simulink model "USART_1_Receive_Send"  (R2018b)
settings: Solver=FixedStepDiscrete  StartTime=0.0  StopTime=10  FixedStep=0.5  RelTol=1e-3  EnableMultiTasking=on
libraries: USART_Lib x6, STM32_Config_Lib x1
settings Model: Creator=reynaudp  LastModifiedBy=bannou
settings DataIOCC: LimitDataPoints=on  SaveFormat=Array  SignalLoggingSaveFormat=ModelDataLogs
settings OptimizationCC: DefaultParameterBehavior=Inlined  DefaultUnderspecifiedDataType=single  LifeSpan=1
settings DebuggingCC: UnderspecifiedInitializationDetection=Classic  MergeDetectMultiDrivingBlocksExec=none  SolverPrmCheckMsg=warning  MultiTaskDSMMsg=warning  MultiTaskCondExecSysMsg=none  AllowSymbolicDim=off  SFUnexpectedBacktrackingDiag=warning  SFNoUnconditionalDefaultTransitionDiag=warning  SFExecutionAtInitializationDiag=none
settings HardwareCC: ProdBitPerPointer=32  ProdBitPerSizeT=32  ProdBitPerPtrDiffT=32  ProdLargestAtomicInteger=Integer  ProdWordSize=32  ProdHWDeviceType=STMicroelectronics->STM32 32-bit Cortex-M
settings ModelReferenceCC: PropagateSignalLabelsOutOfModel=off
settings SFSimCC: SimUseLocalCustomCode=off  CompileTimeRecursionLimit=0  MATLABDynamicMemAlloc=off
settings RTWCC: SystemTargetFile=stm32.tlc  TemplateMakefile=stm32.tmf  Description=stm32 (Embedded Target)  RTWUseLocalCustomCode=off
settings CodeAppCC: IgnoreCustomStorageClasses=off  SimulinkDataObjDesc=on  CustomSymbolStrType=$N$R$M  InsertBlockDesc=on
settings STFCustomTargetCC: CodeReplacementLibrary=ARM CMSIS SIN COS  ParMdlRefBuildCompliant=on  IncludeMdlTerminateFcn=off  CombineOutputUpdateFcns=on  ERTCustomFileBanners=on  SupportNonFinite=off  SupportComplex=off  SupportContinuousTime=off  SupportNonInlinedSFcns=off  RemoveResetFunc=on  SupportVariableSizeSignals=on  MATLABClassNameForMDSCustomization=Simulink.SoftwareTarget.ERTCustomization  SystemTargetFile=stm32.tlc
settings ERTTargetCC: CodeReplacementLibrary=ARM CMSIS SIN COS  MultiwordLength=2048  CompOptLevelCompliant=off  ConcurrentExecutionCompliant=off  IncludeMdlTerminateFcn=off  SupportNonFinite=off  SupportComplex=off  SupportVariableSizeSignals=on  ModelStepFunctionPrototypeControlCompliant=off  CPPClassGenCompliant=off  UseToolchainInfoCompliant=off  ERTSrcFileBannerTemplate=sourceFileTemplate.cgt  ERTHdrFileBannerTemplate=sourceFileTemplate.cgt  ERTDataSrcFileTemplate=sourceFileTemplate.cgt  ERTDataHdrFileTemplate=sourceFileTemplate.cgt  ERTCustomFileTemplate=customRoutineProcess.tlc  ConvertIfToSwitch=off  SuppressUnreachableDefaultCases=off
settings ConfigComp: CovMetricSettings=dw  CovHtmlReporting=on  CovSaveCumulativeToWorkspaceVar=on  CovSaveSingleToWorkspaceVar=on  CovExternalEMLEnable=off  CovSFcnEnable=off

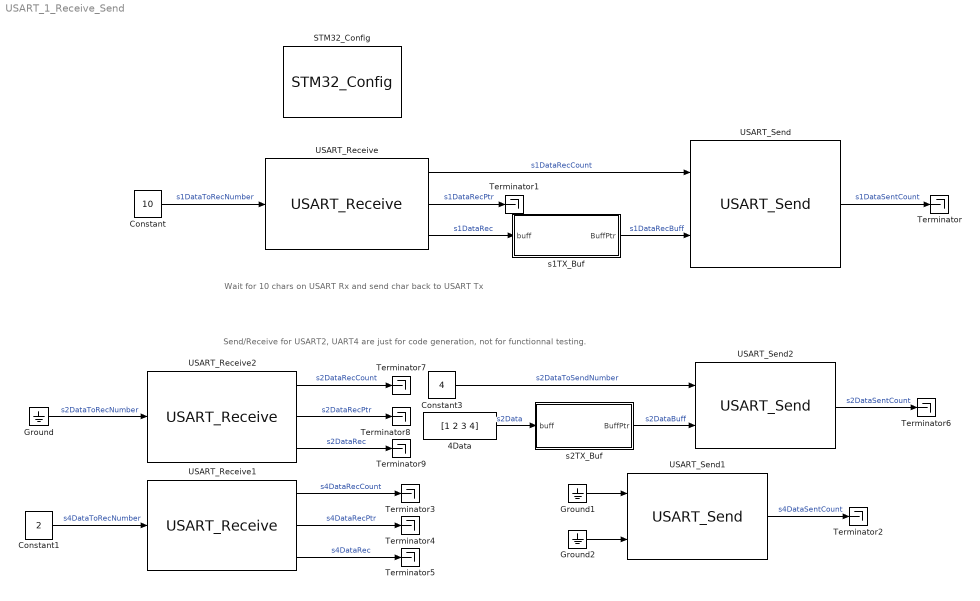
== system USART_1_Receive_Send ==
  note: Send/Receive for USART2, UART4 are just for code generation, not for functionnal testing.
  note: Wait for 10 chars on USART Rx and send char back to USART Tx
  4Data : Constant  Value=[1 2 3 4]  OutDataTypeStr=uint8
  Constant : Constant  Value=10  OutDataTypeStr=uint16
  Constant1 : Constant  Value=2  OutDataTypeStr=uint16
  Constant3 : Constant  Value=4  OutDataTypeStr=uint16
  Ground : Ground
  Ground1 : Ground
  Ground2 : Ground
  STM32_Config : STM32_Config_Lib/STM32_Config  Priority=0  Project_Path=.\  Config_File=USART_1_Receive_Send.ioc  MCU_Name=STM32F429ZITx
      settings: SourceProductName=Target Support Package - STM32 Adapter
  Terminator{,1..9} (10 alike) : Terminator
  USART_Receive : USART_Lib/USART_Receive  USART_name=USART1  Buff_size=32  nbUsart=3  Soft_it=off  Soft_num=0  usartMode=Asynchronous  usartDma_Rx=off  usartDma_Tx=off  usartIt=on
      settings: SourceProductName=Target Support Package - STM32 Adapter
  USART_Receive1 : USART_Lib/USART_Receive  USART_name=UART4  Buff_size=32  nbUsart=3  Soft_it=off  Soft_num=0  usartMode=Asynchronous  usartDma_Rx=off  usartDma_Tx=off  usartIt=on
      settings: SourceProductName=Target Support Package - STM32 Adapter
  USART_Receive2 : USART_Lib/USART_Receive  USART_name=USART2  Buff_size=32  nbUsart=3  Soft_it=off  Soft_num=0  usartMode=Synchronous  usartDma_Rx=off  usartDma_Tx=off  usartIt=on
      settings: SourceProductName=Target Support Package - STM32 Adapter
  USART_Send : USART_Lib/USART_Send  USART_name=USART1  Buff_size=32  nbUsart=3  usartMode=Asynchronous  usartDma_Rx=off  usartDma_Tx=off  usartIt=on
      settings: SourceProductName=Target Support Package - STM32 Adapter
  USART_Send1 : USART_Lib/USART_Send  USART_name=UART4  Buff_size=512  nbUsart=3  usartMode=Asynchronous  usartDma_Rx=off  usartDma_Tx=off  usartIt=on
      settings: SourceProductName=Target Support Package - STM32 Adapter
  USART_Send2 : USART_Lib/USART_Send  USART_name=USART2  Buff_size=512  nbUsart=3  usartMode=Synchronous  usartDma_Rx=off  usartDma_Tx=off  usartIt=on
      settings: SourceProductName=Target Support Package - STM32 Adapter
  s1TX_Buf : MATLAB Function  TreatAsAtomicUnit=on
  s2TX_Buf : MATLAB Function  TreatAsAtomicUnit=on
  wires:
  Constant/1 -> USART_Receive/1  "s1DataToRecNumber"
  s1TX_Buf/1(BuffPtr) -> USART_Send/2  "s1DataRecBuff"
  USART_Receive/3 -> s1TX_Buf/1(buff)  "s1DataRec"
  USART_Receive/1 -> USART_Send/1  "s1DataRecCount"
  USART_Send/1 -> Terminator/1  "s1DataSentCount"
  USART_Receive/2 -> Terminator1/1  "s1DataRecPtr"
  USART_Send1/1 -> Terminator2/1  "s4DataSentCount"
  USART_Receive1/1 -> Terminator3/1  "s4DataRecCount"
  USART_Receive1/2 -> Terminator4/1  "s4DataRecPtr"
  USART_Receive1/3 -> Terminator5/1  "s4DataRec"
  Constant1/1 -> USART_Receive1/1  "s4DataToRecNumber"
  Ground1/1 -> USART_Send1/1
  Ground2/1 -> USART_Send1/2
  Constant3/1 -> USART_Send2/1  "s2DataToSendNumber"
  USART_Send2/1 -> Terminator6/1  "s2DataSentCount"
  4Data/1 -> s2TX_Buf/1(buff)  "s2Data"
  s2TX_Buf/1(BuffPtr) -> USART_Send2/2  "s2DataBuff"
  USART_Receive2/2 -> Terminator8/1  "s2DataRecPtr"
  USART_Receive2/3 -> Terminator9/1  "s2DataRec"
  Ground/1 -> USART_Receive2/1  "s2DataToRecNumber"
  USART_Receive2/1 -> Terminator7/1  "s2DataRecCount"

== matlab function USART_1_Receive_Send/s2TX_Buf ==
  data: BuffPtr output uint32 size=1; buff input
function BuffPtr = convert(buff)
if coder.target('Sfun')
    % Executing in MATLAB, Buff is null
    BuffPtr = uint32(0);
    %NbChar = uint16(0);
else
    coder.cinclude('getBuffPtr.h');
    % Executing in the generated code.
    BuffPtr = coder.ceval('getBuffPtr',coder.rref(buff));
end
end

== matlab function USART_1_Receive_Send/s1TX_Buf ==
  data: BuffPtr output uint32 size=1; buff input
function BuffPtr = convert(buff)
if coder.target('Sfun')
    % Executing in MATLAB, Buff is null
    BuffPtr = uint32(0);
    %NbChar = uint16(0);
else
    coder.cinclude('getBuffPtr.h');
    % Executing in the generated code.
    BuffPtr = coder.ceval('getBuffPtr',coder.rref(buff));
end
end
